simulink model "SOP_limiter"  (R2024a)
settings: Solver=VariableStepAuto  StartTime=0.0  StopTime=10.0  RelTol=1e-3
undefined symbols (not defined in the file or in its folder): CONT_CHARGE_LIMIT_I, CONT_CHARGE_LIMIT_SOC, CONT_CHARGE_LIMIT_T, DiscIntNeverNeededParam, magnitude, MAX_CURRENT_LIMIT, SOP_TIMESTEP, Vmax
settings Model: Creator=mmackenzie  LastModifiedBy=mmackenzie

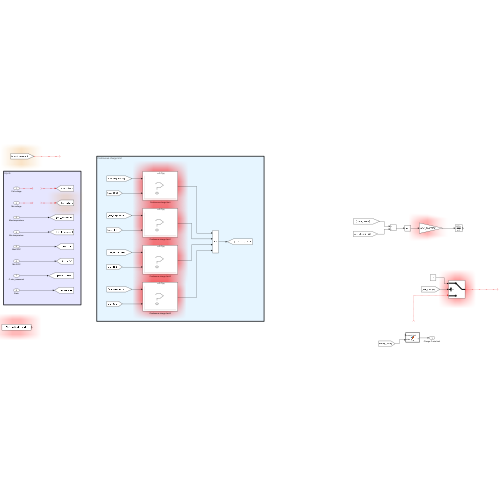
[thumbnail: Simulink's stored preview of the top-level diagram]
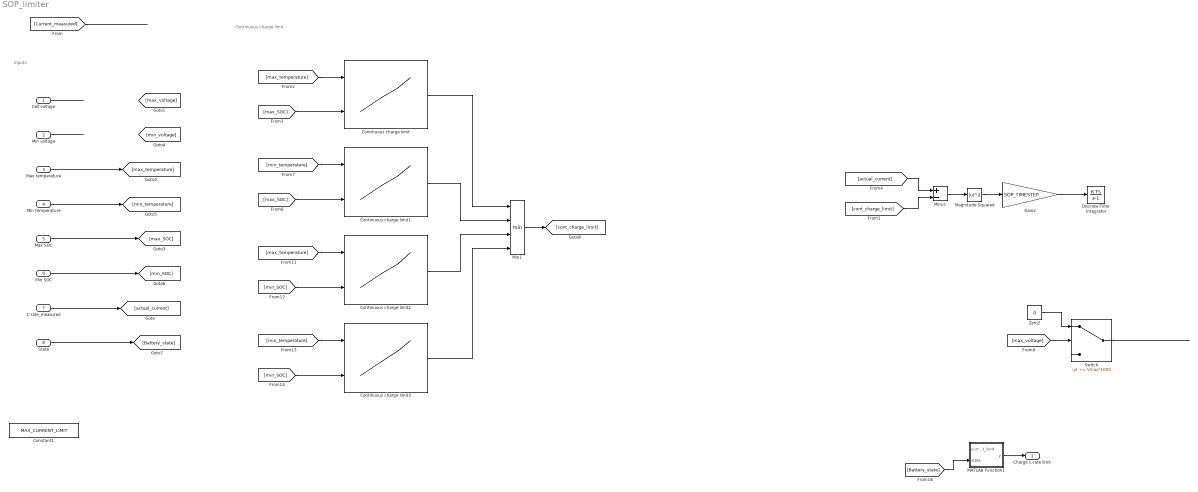
== system SOP_limiter ==
  note: Inputs
  note: Continuous charge limit
  Cell voltage : Inport
  Min voltage : Inport  Port=2
  Max temperature : Inport  Port=3
  Min temperature : Inport  Port=4
  Max SOC : Inport  Port=5
  Min SOC : Inport  Port=6
  C-rate_measured : Inport  Port=7
  State : Inport  Port=8
  Constant1 : Constant  Value=MAX_CURRENT_LIMIT
  Continuous charge limit{,1..3} (4 alike) : Lookup_n-D  BreakpointsForDimension1=CONT_CHARGE_LIMIT_T  BreakpointsForDimension2=CONT_CHARGE_LIMIT_SOC  Table=CONT_CHARGE_LIMIT_I  ExtrapMethod=Clip  InternalRulePriority=Speed  RndMeth=Simplest
      settings: InputPortMap=u0,u1
  Discrete-Time Integrator : DiscreteIntegrator  SampleTime=-1  ICPrevOutput=DiscIntNeverNeededParam  ICPrevScaledInput=DiscIntNeverNeededParam
  Gain2 : Gain  Gain=SOP_TIMESTEP
  MATLAB Function1 : MATLAB Function  TreatAsAtomicUnit=on
  Magnitude Squared : Math  Operator=magnitude^2
  Min1 : MinMax  Inputs=4
  Minus : Sum  Inputs=+-
  Switch : Switch  Threshold=Vmax*1000  SaturateOnIntegerOverflow=off  InputSameDT=off
  Zero2 : Constant  Value=0  OutDataTypeStr=Inherit: Inherit via back propagation
  Charge C-rate limit : Outport
  wires:
  [Battery_state] -> MATLAB Function1/2(state)
  ? -> [min_voltage]
  [max_temperature] -> Continuous charge limit/1
  State/1 -> [Battery_state]
  Min temperature/1 -> [min_temperature]
  ? -> [max_voltage]
  Max temperature/1 -> [max_temperature]
  Continuous charge limit/1 -> Min1/1
  MATLAB Function1/1(y) -> Charge C-rate limit/1
  [max_SOC] -> Continuous charge limit1/2
  Min voltage/1 -> ?
  C-rate_measured/1 -> [actual_current]
  [Current_measured] -> ?
  Min SOC/1 -> [min_SOC]
  [max_SOC] -> Continuous charge limit/2
  [min_temperature] -> Continuous charge limit1/1
  Max SOC/1 -> [max_SOC]
  Cell voltage/1 -> ?
  Switch/1 -> ?
  Zero2/1 -> Switch/1
  [max_voltage] -> Switch/2
  ? -> Switch/3
  [min_temperature] -> Continuous charge limit3/1
  [min_SOC] -> Continuous charge limit2/2
  [min_SOC] -> Continuous charge limit3/2
  [max_temperature] -> Continuous charge limit2/1
  Continuous charge limit1/1 -> Min1/2
  Continuous charge limit2/1 -> Min1/3
  Continuous charge limit3/1 -> Min1/4
  Min1/1 -> [cont_charge_limit]
  [cont_charge_limit] -> Minus/2
  [actual_current] -> Minus/1
  Minus/1 -> Magnitude Squared/1
  Magnitude Squared/1 -> Gain2/1
  Gain2/1 -> Discrete-Time Integrator/1

== matlab function SOP_limiter/MATLAB Function1 ==
  data: current_limit input; y output; state input
function y = fcn(current_limit, state)
if state == "CHARGE"
    y = current_limit;
else
    y = 0;
end
